simulink model "A06_L9_4"  (R2016b)
settings: Solver=ode45  StartTime=0.0  StopTime=10.0  RelTol=1e-3  EnableMultiTasking=on
settings Model: Creator=User  LastModifiedBy=mluser
settings DataIOCC: LimitDataPoints=on  SaveFormat=Array
settings OptimizationCC: LifeSpan=inf
settings DebuggingCC: SolverPrmCheckMsg=warning  SFUnexpectedBacktrackingDiag=warning  SFNoUnconditionalDefaultTransitionDiag=warning  SFExecutionAtInitializationDiag=none
settings HardwareCC: ProdBitPerPointer=32  ProdBitPerSizeT=32  ProdBitPerPtrDiffT=32  ProdLargestAtomicFloat=None  ProdIntDivRoundTo=Undefined  ProdEndianess=Unspecified  ProdWordSize=32  ProdHWDeviceType=32-bit Generic
settings ModelReferenceCC: PropagateSignalLabelsOutOfModel=off
settings GRTTargetCC: TargetLangStandard=C89/C90 (ANSI)
settings ConfigComp: CovMetricSettings=dw  CovSaveCumulativeToWorkspaceVar=on  CovSaveSingleToWorkspaceVar=on  CovExternalEMLEnable=off  CovSFcnEnable=off

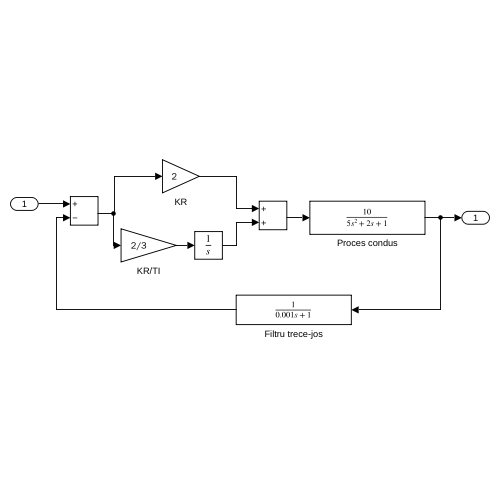
[thumbnail: Simulink's stored preview of the top-level diagram]
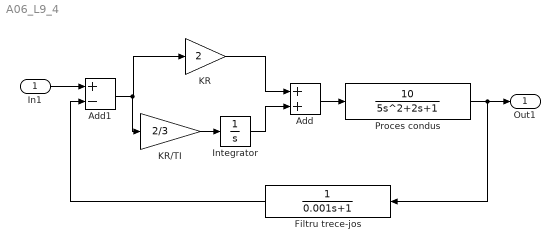
== system A06_L9_4 ==
  In1 : Inport
  Add : Sum
  Add1 : Sum  Inputs=+-
  Filtru trece-jos : TransferFcn  Denominator=[0.001 1]
  Integrator : Integrator
  KR : Gain  Gain=2
  KR/TI : Gain  Gain=2/3
  Proces condus : TransferFcn  Numerator=[10]  Denominator=[5 2 1]
  Out1 : Outport
  wires:
  Add/1 -> Proces condus/1
  KR/1 -> Add/1
  Integrator/1 -> Add/2
  KR/TI/1 -> Integrator/1
  Proces condus/1 -> Out1/1, Filtru trece-jos/1
  Add1/1 -> KR/TI/1, KR/1
  In1/1 -> Add1/1
  Filtru trece-jos/1 -> Add1/2
